simulink model "pureController"  (R2019a)
settings: Solver=FixedStepAuto  StartTime=0.0  StopTime=10  FixedStep=0.01  RelTol=1e-3
values from neighbouring files (symbols this model uses):
  k = 0    [main.m]    (also in pure_controller.m = 0.1)
  lookaheadDistance = 0.25    [main.m]
  ref_poses = [cx,cy]    [main.m]
  Target_Speed = 1    [main.m]
  WheelBase = 0.3    [main.m]
libraries: simulink_extras x4, autolibshared x1
settings Model: Creator=Li Fang  LastModifiedBy=Li Fang

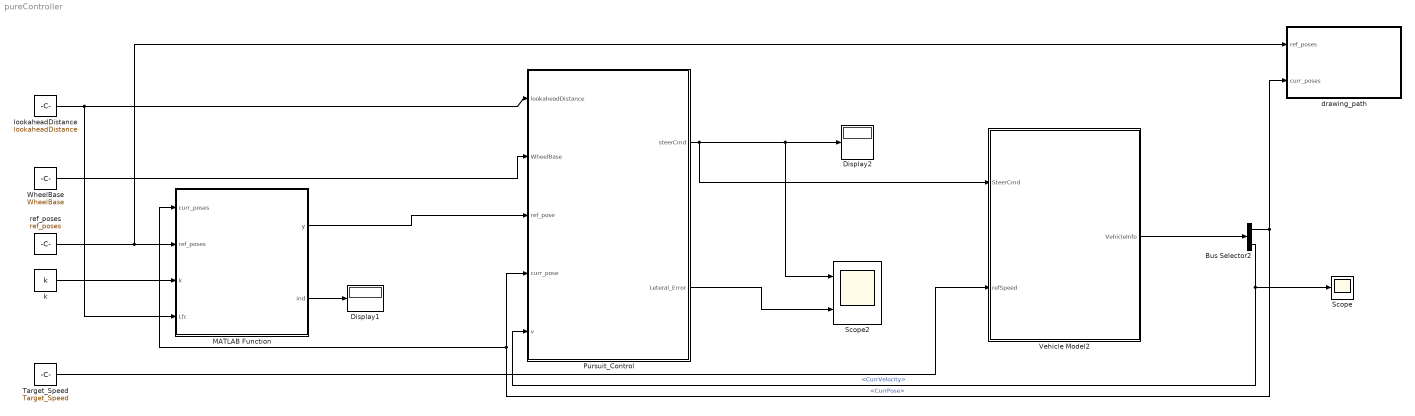
== system pureController ==
  Bus Selector2 : BusSelector  OutputSignals=CurrPose,CurrVelocity
  Display1 : Display
  Display2 : Display
  MATLAB Function : MATLAB Function  TreatAsAtomicUnit=on
  Pursuit_Control : Subsystem
  Scope : Scope
  Scope2 : Scope  NumInputPorts=2
  Target_Speed : Constant  Value=Target_Speed
  Vehicle Model2 : Subsystem
  WheelBase : Constant  Value=WheelBase
  drawing_path : MATLAB Function  TreatAsAtomicUnit=on
  k : Constant  Value=k
  lookaheadDistance : Constant  Value=lookaheadDistance
  ref_poses : Constant  Value=ref_poses
  wires:
  lookaheadDistance/1 -> MATLAB Function/4(Lfc), Pursuit_Control/1(lookaheadDistance)
  MATLAB Function/1(y) -> Pursuit_Control/3(ref_pose)
  Pursuit_Control/2(Leteral_Error) -> Scope2/2
  k/1 -> MATLAB Function/3(k)
  Vehicle Model2/1(VehicleInfo) -> Bus Selector2/1
  Target_Speed/1 -> Vehicle Model2/2(refSpeed)
  WheelBase/1 -> Pursuit_Control/2(WheelBase)
  Pursuit_Control/1(steerCmd) -> Vehicle Model2/1(SteerCmd), Scope2/1, Display2/1
  Bus Selector2/2 -> Pursuit_Control/5(v), Scope/1  "<CurrVelocity>"
  MATLAB Function/2(ind) -> Display1/1
  ref_poses/1 -> drawing_path/1(ref_poses), MATLAB Function/2(ref_poses)
  Bus Selector2/1 -> Pursuit_Control/4(curr_pose), MATLAB Function/1(curr_poses), drawing_path/2(curr_poses)  "<CurrPose>"

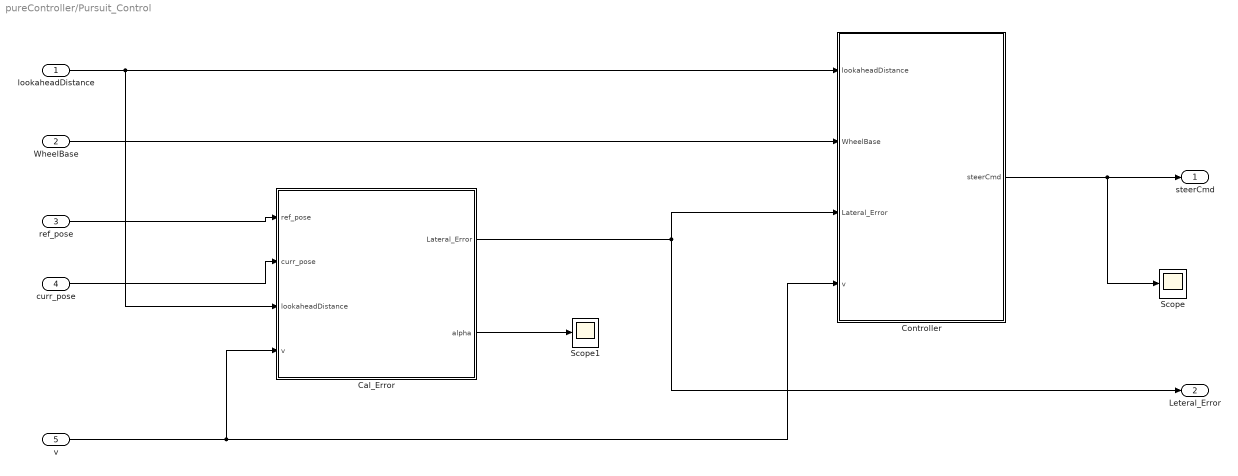
== system pureController/Pursuit_Control ==
  lookaheadDistance : Inport
  WheelBase : Inport  Port=2
  ref_pose : Inport  Port=3
  curr_pose : Inport  Port=4
  v : Inport  Port=5
  Cal_Error : Subsystem
  Controller : Subsystem
  Scope : Scope
  Scope1 : Scope
  steerCmd : Outport
  Leteral_Error : Outport  Port=2
  wires:
  curr_pose/1 -> Cal_Error/2(curr_pose)
  Cal_Error/1(Lateral_Error) -> Leteral_Error/1, Controller/3(Lateral_Error)
  lookaheadDistance/1 -> Controller/1(lookaheadDistance), Cal_Error/3(lookaheadDistance)
  ref_pose/1 -> Cal_Error/1(ref_pose)
  WheelBase/1 -> Controller/2(WheelBase)
  Controller/1(steerCmd) -> Scope/1, steerCmd/1
  v/1 -> Controller/4(v), Cal_Error/4(v)
  Cal_Error/2(alpha) -> Scope1/1

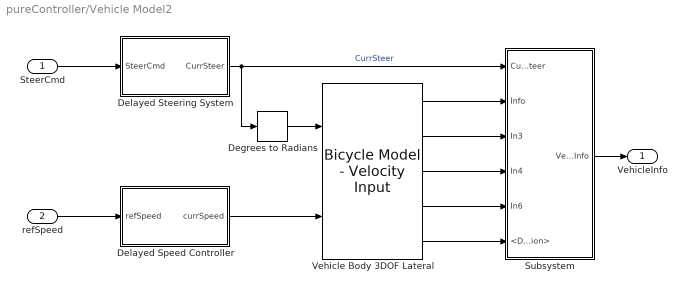
== system pureController/Vehicle Model2 ==
  SteerCmd : Inport
  refSpeed : Inport  Port=2
  Degrees to Radians : simulink_extras/Transformations/Degrees to Radians
  Delayed Speed Controller : Subsystem
  Delayed Steering System : Subsystem
  Subsystem : Subsystem
  Vehicle Body 3DOF Lateral : autolibshared/Bicycle Model - Velocity Input  trackMode=Single (bicycle)  inputMode=External longitudinal forces  frontSteerMode=on  rearSteerMode=off  windMode=off  muMode=off  extFMode=off  extMMode=off  aMode=3  NF=2  NR=2  m=1.2  a=0.2  b=0.1  h=0.04  X_o=0  xdot_o=0  CalphaMode=off  sigmaMode=on  w=[1.4,1.4]  Cy_f=19e3  Cy_r=20e3  sigma_f=.1  sigma_r=.1  alpha_f_brk=[-.1 .1]  Cy_f_data=[-9e3 9e3]  alpha_r_brk=[-.1 .1]  Cy_r_data=[-9e3 9e3]  Y_o=0.3  ydot_o=0  Izz=0.004  psi_o=deg2rad(0)  r_o=0  Af=2  Cd=.3  Cl=.1  Cpm=.1  beta_w=[0:0.01:0.3]  Cs=[0:0.03:0.9]  Cym=[0:0.01:0.3]  Pabs=101325  Tair=273  g=9.81  mu=1  xdot_tol=0.01  Fznom=5000  Fxtire_sat=1e6  Fytire_sat=1e6  longOff=0  latOff=0  vertOff=0
      settings: SourceProductName=Powertrain Blockset  SourceProductBaseCode=PW
  VehicleInfo : Outport
  wires:
  Delayed Speed Controller/1(currSpeed) -> Vehicle Body 3DOF Lateral/2
  Degrees to Radians/1 -> Vehicle Body 3DOF Lateral/1
  Delayed Steering System/1(CurrSteer) -> Subsystem/1(CurrSteer), Degrees to Radians/1  "CurrSteer"
  SteerCmd/1 -> Delayed Steering System/1(SteerCmd)
  Subsystem/1(VehicleInfo) -> VehicleInfo/1
  Vehicle Body 3DOF Lateral/1 -> Subsystem/2(Info)
  Vehicle Body 3DOF Lateral/2 -> Subsystem/3(In3)
  Vehicle Body 3DOF Lateral/3 -> Subsystem/4(In4)
  Vehicle Body 3DOF Lateral/4 -> Subsystem/5(In6)
  Vehicle Body 3DOF Lateral/5 -> Subsystem/6(<Direction>)
  refSpeed/1 -> Delayed Speed Controller/1(refSpeed)

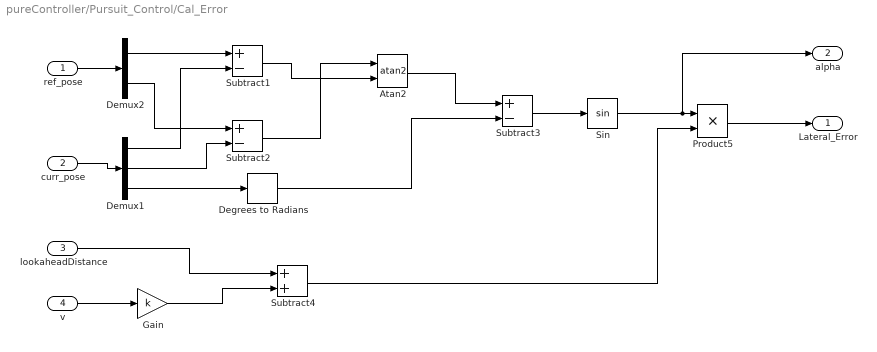
== system pureController/Pursuit_Control/Cal_Error ==
  ref_pose : Inport
  curr_pose : Inport  Port=2
  lookaheadDistance : Inport  Port=3
  v : Inport  Port=4
  Atan2 : Trigonometry  Operator=atan2
  Degrees to Radians : simulink_extras/Transformations/Degrees to Radians
  Demux1 : Demux  Outputs=3
  Demux2 : Demux  Outputs=2
  Gain : Gain  Gain=k
  Product5 : Product
  Sin : Trigonometry
  Subtract1 : Sum  Inputs=+-
  Subtract2 : Sum  Inputs=+-
  Subtract3 : Sum  Inputs=+-
  Subtract4 : Sum
  Lateral_Error : Outport
  alpha : Outport  Port=2
  wires:
  Demux1/1 -> Subtract1/2
  Demux2/2 -> Subtract2/1
  curr_pose/1 -> Demux1/1
  Demux1/2 -> Subtract2/2
  Product5/1 -> Lateral_Error/1
  ref_pose/1 -> Demux2/1
  Subtract3/1 -> Sin/1
  Sin/1 -> alpha/1, Product5/1
  Demux2/1 -> Subtract1/1
  Atan2/1 -> Subtract3/1
  Subtract2/1 -> Atan2/1
  Subtract1/1 -> Atan2/2
  Demux1/3 -> Degrees to Radians/1
  Degrees to Radians/1 -> Subtract3/2
  lookaheadDistance/1 -> Subtract4/1
  Gain/1 -> Subtract4/2
  v/1 -> Gain/1
  Subtract4/1 -> Product5/2

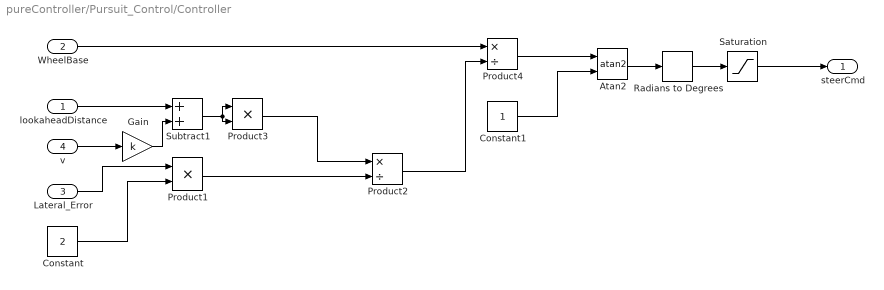
== system pureController/Pursuit_Control/Controller ==
  lookaheadDistance : Inport
  WheelBase : Inport  Port=2
  Lateral_Error : Inport  Port=3
  v : Inport  Port=4
  Atan2 : Trigonometry  Operator=atan2
  Constant : Constant  Value=2
  Constant1 : Constant
  Gain : Gain  Gain=k
  Product1 : Product
  Product2 : Product  Inputs=*/
  Product3 : Product  Inputs=**
  Product4 : Product  Inputs=*/
  Radians to Degrees : simulink_extras/Transformations/Radians to Degrees
  Saturation : Saturate  UpperLimit=35  LowerLimit=-35
  Subtract1 : Sum
  steerCmd : Outport
  wires:
  Radians to Degrees/1 -> Saturation/1
  Product2/1 -> Product4/2
  Constant/1 -> Product1/2
  Product3/1 -> Product2/1
  Product1/1 -> Product2/2
  Lateral_Error/1 -> Product1/1
  WheelBase/1 -> Product4/1
  Saturation/1 -> steerCmd/1
  Product4/1 -> Atan2/1
  Atan2/1 -> Radians to Degrees/1
  v/1 -> Gain/1
  Gain/1 -> Subtract1/2
  lookaheadDistance/1 -> Subtract1/1
  Subtract1/1 -> Product3/2, Product3/1
  Constant1/1 -> Atan2/2

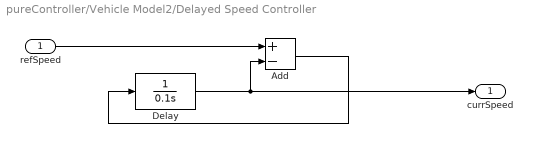
== system pureController/Vehicle Model2/Delayed Speed Controller ==
  refSpeed : Inport
  Add : Sum  Inputs=+-
  Delay : TransferFcn  Denominator=[0.1 0]
  currSpeed : Outport
  wires:
  Add/1 -> Delay/1
  refSpeed/1 -> Add/1
  Delay/1 -> currSpeed/1, Add/2

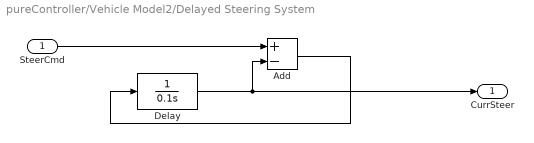
== system pureController/Vehicle Model2/Delayed Steering System ==
  SteerCmd : Inport
  Add : Sum  Inputs=+-
  Delay : TransferFcn  Denominator=[0.1 0]
  CurrSteer : Outport
  wires:
  Add/1 -> Delay/1
  SteerCmd/1 -> Add/1
  Delay/1 -> CurrSteer/1, Add/2

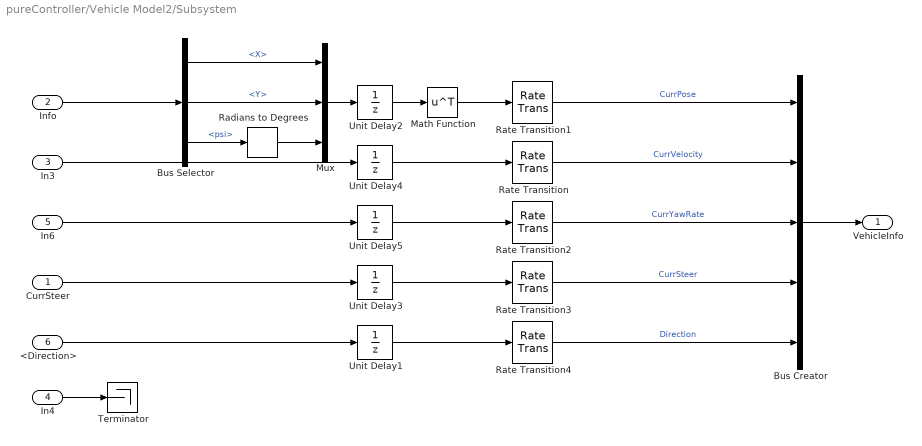
== system pureController/Vehicle Model2/Subsystem ==
  CurrSteer : Inport
  Info : Inport  Port=2
  In3 : Inport  Port=3
  In4 : Inport  Port=4
  In6 : Inport  Port=5
  <Direction> : Inport  Port=6
  Bus Creator : BusCreator  Inputs=5
  Bus Selector : BusSelector  OutputSignals=InertFrm.RearAxl.Disp.X,InertFrm.RearAxl.Disp.Y,InertFrm.Cg.Ang.psi
  Math Function : Math  Operator=transpose  SaturateOnIntegerOverflow=on
  Mux : Mux  Inputs=3
  Radians to Degrees : simulink_extras/Transformations/Radians to Degrees
  Rate Transition : RateTransition  OutPortSampleTime=0.01
  Rate Transition1 : RateTransition  InitialCondition=[0,0.3,0]  OutPortSampleTime=0.01
  Rate Transition2 : RateTransition  OutPortSampleTime=0.01
  Rate Transition3 : RateTransition  OutPortSampleTime=0.01
  Rate Transition4 : RateTransition  InitialCondition=1  OutPortSampleTime=0.01
  Terminator : Terminator
  Unit Delay1 : UnitDelay  InitialCondition=1  SampleTime=-1  HasFrameUpgradeWarning=on
  Unit Delay2 : UnitDelay  InitialCondition=[0,0.3,0]  SampleTime=-1  HasFrameUpgradeWarning=on
  Unit Delay3 : UnitDelay  SampleTime=-1  HasFrameUpgradeWarning=on
  Unit Delay4 : UnitDelay  SampleTime=-1  HasFrameUpgradeWarning=on
  Unit Delay5 : UnitDelay  SampleTime=-1  HasFrameUpgradeWarning=on
  VehicleInfo : Outport
  wires:
  Unit Delay1/1 -> Rate Transition4/1
  CurrSteer/1 -> Unit Delay3/1
  Unit Delay5/1 -> Rate Transition2/1
  <Direction>/1 -> Unit Delay1/1
  Unit Delay4/1 -> Rate Transition/1
  Math Function/1 -> Rate Transition1/1
  Rate Transition/1 -> Bus Creator/2  "CurrVelocity"
  Unit Delay3/1 -> Rate Transition3/1
  Rate Transition3/1 -> Bus Creator/4  "CurrSteer"
  Rate Transition1/1 -> Bus Creator/1  "CurrPose"
  Rate Transition2/1 -> Bus Creator/3  "CurrYawRate"
  Rate Transition4/1 -> Bus Creator/5  "Direction"
  Unit Delay2/1 -> Math Function/1
  Info/1 -> Bus Selector/1
  Radians to Degrees/1 -> Mux/3
  Bus Selector/2 -> Mux/2  "<Y>"
  Bus Selector/1 -> Mux/1  "<X>"
  Mux/1 -> Unit Delay2/1
  In3/1 -> Unit Delay4/1
  In4/1 -> Terminator/1
  In6/1 -> Unit Delay5/1
  Bus Selector/3 -> Radians to Degrees/1  "<psi>"
  Bus Creator/1 -> VehicleInfo/1

== matlab function pureController/MATLAB Function ==
  data: curr_poses input; y output; ref_poses input; k input; Lfc input; ind output
function [y,ind] = find_target_index(curr_poses, ref_poses,k,Lfc)
    N =  length(ref_poses);                                     %N = 501
    Distance = zeros(N,1);                               % 501行 1列的矩阵
    for i = 1:N
    %Distance(i) =  sqrt((ref_poses(i,1)-curr_poses(1,1))^2 + (ref_poses(i,2)-curr_poses(1,2))^2);%每一个预瞄点到初始位置的距离
        Distance(i) = norm(curr_poses(1,1:2)-ref_poses(i,1:2));
    end

    [~, location]= min(Distance);                        %找出最近的距离对应的位置
    ind = location;
    L=0;
 %   Lf = 0.15;
    Lf = k*curr_poses(1,3)+Lfc;
    while Lf>L && (ind+1)<length(ref_poses)
%        dx = ref_poses(ind+1,1) - ref_poses(ind,1);
%        dy = ref_poses(ind+1,2) - ref_poses(ind,2);
%        L = L + sqrt(dx^2+dy^2);
        L = norm(curr_poses(1,1:2)-ref_poses(ind,1:2));
        ind= ind + 1;
    end
    f = ref_poses(ind,1:2);
    y=f';
end

== matlab function pureController/drawing_path ==
  data: ref_poses input; curr_poses input
function drawing_path(ref_poses,curr_poses)
    cx = ref_poses(:,1);
    cy = ref_poses(:,2);
    x = curr_poses(1,1);
    y = curr_poses(1,2);
        % pause(0.1)
    plot(cx,cy,'g',x,y,'ro')        %将预瞄点位置用蓝色表示，当前位置用红色表示
    drawnow
    hold on

end
